simulink model "Joystick_Demo"  (R2018a)
settings: Solver=FixedStepAuto  StartTime=0.0  StopTime=inf  FixedStep=.25  RelTol=1e-3  EnableMultiTasking=on
libraries: simulink x5, arduinolib x5
settings Model: SimulationMode=external  ExtModeTrigDuration=2  Creator=jonathancoulter  LastModifiedBy=jonathancoulter
settings SolverCC: AutoInsertRateTranBlk=on
settings OptimizationCC: UseFloatMulNetSlope=on  PassReuseOutputArgsThreshold=0  EfficientFloat2IntCast=on  MaxStackSize=64
settings DebuggingCC: ParameterTunabilityLossMsg=error
settings HardwareCC: ProdBitPerInt=16  ProdBitPerPointer=16  ProdBitPerSizeT=16  ProdBitPerPtrDiffT=16  ProdLargestAtomicFloat=None  ProdWordSize=8  ProdHWDeviceType=Atmel->AVR  UseEmbeddedCoderFeatures=off
settings ModelReferenceCC: ModelReferenceMinAlgLoopOccurrences=on
settings SFSimCC: MATLABDynamicMemAlloc=off
settings RTWCC: SystemTargetFile=ert.tlc  HardwareBoard=Arduino Mega 2560  TLCOptions=-aInlineSetEventsForThisBaseRateFcn=TLC_FALSE -aSuppressMultiTaskScheduler=TLC_FALSE -aRateBasedStepFcn=1  TemplateMakefile=ert_default_tmf  Toolchain=Arduino AVR  BuildConfiguration=Faster Runs  CheckMdlBeforeBuild=Warning
settings CodeAppCC: ForceParamTrailComments=on  OperatorAnnotations=on  StateflowObjectComments=on  MATLABSourceComments=on
settings ERTTargetCC: ERTCustomFileBanners=off  SupportContinuousTime=on  SupportNonInlinedSFcns=on  RemoveResetFunc=off  SupportVariableSizeSignals=on  ModelStepFunctionPrototypeControlCompliant=off

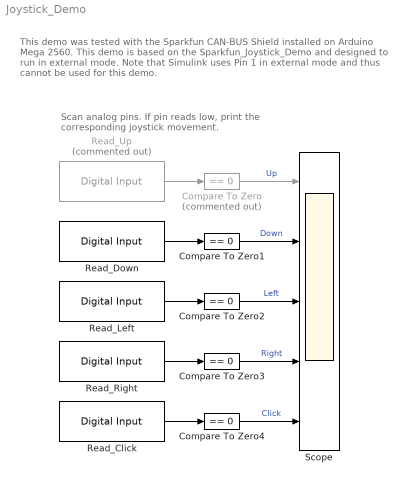
== system Joystick_Demo ==
  note: This demo was tested with the Sparkfun CAN-BUS Shield installed on Arduino Mega 2560.
      | This demo is based on the Sparkfun_Joystick_Demo and designed to run in external mode.
      | Note that Simulink uses Pin 1 in external mode and thus cannot be used for this demo.
  note: Scan analog pins. If pin reads low, print the corresponding joystick movement.
  Compare To Zero : simulink/Logic and Bit Operations/Compare To Zero  Commented=on  relop===  OutDataTypeStr=boolean
  Compare To Zero{1..4} (4 alike) : simulink/Logic and Bit Operations/Compare To Zero  relop===  OutDataTypeStr=boolean
  Read_Click : arduinolib/Digital Input  pinNumber=4  sampleTime=-1  blockPlatform=arduino
      settings: SourceProductName=Simulink Support Package for Arduino Hardware
  Read_Down : arduinolib/Digital Input  pinNumber=3  sampleTime=-1  blockPlatform=arduino
      settings: SourceProductName=Simulink Support Package for Arduino Hardware
  Read_Left : arduinolib/Digital Input  pinNumber=2  sampleTime=-1  blockPlatform=arduino
      settings: SourceProductName=Simulink Support Package for Arduino Hardware
  Read_Right : arduinolib/Digital Input  pinNumber=5  sampleTime=-1  blockPlatform=arduino
      settings: SourceProductName=Simulink Support Package for Arduino Hardware
  Read_Up : arduinolib/Digital Input  Commented=on  pinNumber=1  sampleTime=-1  blockPlatform=arduino
      settings: SourceProductName=Simulink Support Package for Arduino Hardware
  Scope : Scope  NumInputPorts=5
  wires:
  Read_Up/1 -> Compare To Zero/1
  Compare To Zero/1 -> Scope/1  "Up"
  Read_Left/1 -> Compare To Zero2/1
  Read_Right/1 -> Compare To Zero3/1
  Read_Click/1 -> Compare To Zero4/1
  Read_Down/1 -> Compare To Zero1/1
  Compare To Zero1/1 -> Scope/2  "Down"
  Compare To Zero2/1 -> Scope/3  "Left"
  Compare To Zero3/1 -> Scope/4  "Right"
  Compare To Zero4/1 -> Scope/5  "Click"
